simulink model "E_Platoon_simscape"  (R2025b)
settings: Solver=FixedStepAuto  StartTime=0.0  StopTime=inf  FixedStep=0.01  RelTol=1e-3
values from neighbouring files (symbols this model uses):
  battery_SOC_resistance = battery_SOC(:,3)    [EV_Truck.m]
  battery_SOC_SOC = battery_SOC(:,1)    [EV_Truck.m]
  battery_SOC_voltage = battery_SOC(:,2)    [EV_Truck.m]
  motor_efficiency_efficiency = table2array(motor_efficiency(2:height(motor_efficiency),2:width(motor_efficiency)))    [EV_Truck.m]
  motor_efficiency_RPM = table2array(motor_efficiency(2:height(motor_efficiency),1))    [EV_Truck.m]
  motor_efficiency_torque = transpose(motor_efficiency_torque)    [EV_Truck.m]
  motor_RPM_torque = table2array(motor_torque(1:14,1))    [EV_Truck.m]
  motor_torque_RPM = table2array(motor_torque(1:14,2))    [EV_Truck.m]
undefined symbols (not defined in the file or in its folder): battery_builder_rtmsupport, DiscIntNeverNeededParam, gcbh
libraries: simulink x8, fl_lib x8, nesl_utility x8, Batteries_lib x4, mpcadaslib x2, slpidlib x2
(part 1 of 3)
settings Model: Creator=Administrator  LastModifiedBy=geunu6319
settings SolverCC: AlgebraicLoopSolver=TrustRegion
settings DataIOCC: ExternalInput=EV_ModelingScenario.getElement('Input')  ReturnWorkspaceOutputs=off
settings OptimizationCC: DefaultParameterBehavior=Inlined  UseDivisionForNetSlopeComputation=on  GainParamInheritBuiltInType=on  UseFloatMulNetSlope=on  UseSpecifiedMinMax=on  InlineInvariantSignals=on  PassReuseOutputArgsAs=Individual arguments  ZeroExternalMemoryAtStartup=off  ZeroInternalMemoryAtStartup=off  NoFixptDivByZeroProtection=on  EfficientFloat2IntCast=on  LifeSpan=1  OptimizeBlockOrder=speed  DifferentSizesBufferReuse=on  EfficientTunableParamExpr=on
settings DebuggingCC: ParameterTunabilityLossMsg=error  UnconnectedInputMsg=warning  UnconnectedOutputMsg=warning  UnconnectedLineMsg=warning
settings HardwareCC: TargetBitPerLong=64.0  TargetBitPerPointer=64.0  TargetBitPerSizeT=64.0  TargetBitPerPtrDiffT=64.0  TargetLargestAtomicInteger=LongLong  TargetLargestAtomicFloat=Double  TargetLongLongMode=on  TargetIntDivRoundTo=Zero  TargetEndianess=LittleEndian  TargetWordSize=64.0  TargetHWDeviceType=ARM Compatible->ARM Cortex-A (64-bit)
settings ModelReferenceCC: EnableRefExpFcnMdlSchedulingChecks=on
settings SFSimCC: CompileTimeRecursionLimit=0.0  EnableRuntimeRecursion=off  MATLABDynamicMemAlloc=off  SimTargetLang=C++  SimDLTargetLibrary=mkl-dnn
settings RTWCC: SystemTargetFile=ert.tlc  GenCodeOnly=on  TemplateMakefile=ert_default_tmf  BuildConfiguration=Faster Runs  PortableWordSizes=on  CodeExecutionProfiling=on  CodeProfilingSaveOptions=AllData  CodeProfilingInstrumentation=coarse  DataTypeReplacement=CDataTypesFixedWidth  TargetLang=C++  GPUComputeCapability=3.5  DLArmComputeVersion=19.05  Description=Embedded Coder
settings CodeAppCC: ForceParamTrailComments=on  IgnoreCustomStorageClasses=off  IgnoreTestpoints=on  OperatorAnnotations=on  SimulinkDataObjDesc=on  SFDataObjDesc=on  CustomSymbolStrGlobalVar=rt$N$M  CustomSymbolStrType=$N$M  CustomSymbolStrFcn=$N$M$F  CustomSymbolStrMacro=$N$M  InsertBlockDesc=on
settings ERTTargetCC: RootIOFormat=Structure reference  ERTCustomFileTemplate=example_file_process.tlc  ERTFilePackagingFormat=CompactWithDataFile  SuppressUnreachableDefaultCases=off  MaxIdInt64=INT64_MAX  MinIdInt64=INT64_MIN  MaxIdUint64=UINT64_MAX  MaxIdInt32=INT32_MAX  MinIdInt32=INT32_MIN  MaxIdUint32=UINT32_MAX  MaxIdInt16=INT16_MAX  MinIdInt16=INT16_MIN  MaxIdUint16=UINT16_MAX  MaxIdInt8=INT8_MAX  MinIdInt8=INT8_MIN  MaxIdUint8=UINT8_MAX  TargetLangStandard=C++11 (ISO)  GenerateSampleERTMain=on  IncludeMdlTerminateFcn=off  CombineSignalStateStructs=on  CodeInterfacePackaging=C++ class  SupportComplex=off  SupportContinuousTime=on  SupportNonInlinedSFcns=on  ParenthesesLevel=Standards

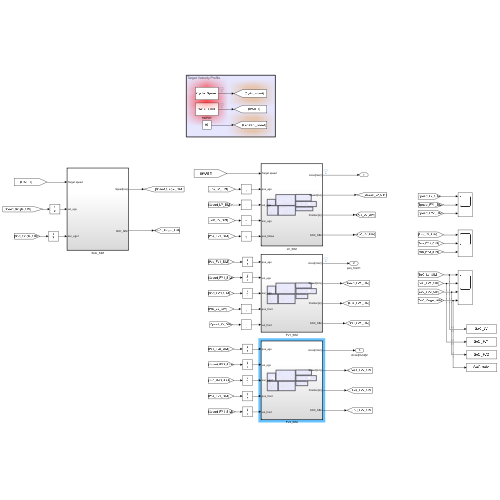
[thumbnail: Simulink's stored preview of the top-level diagram]
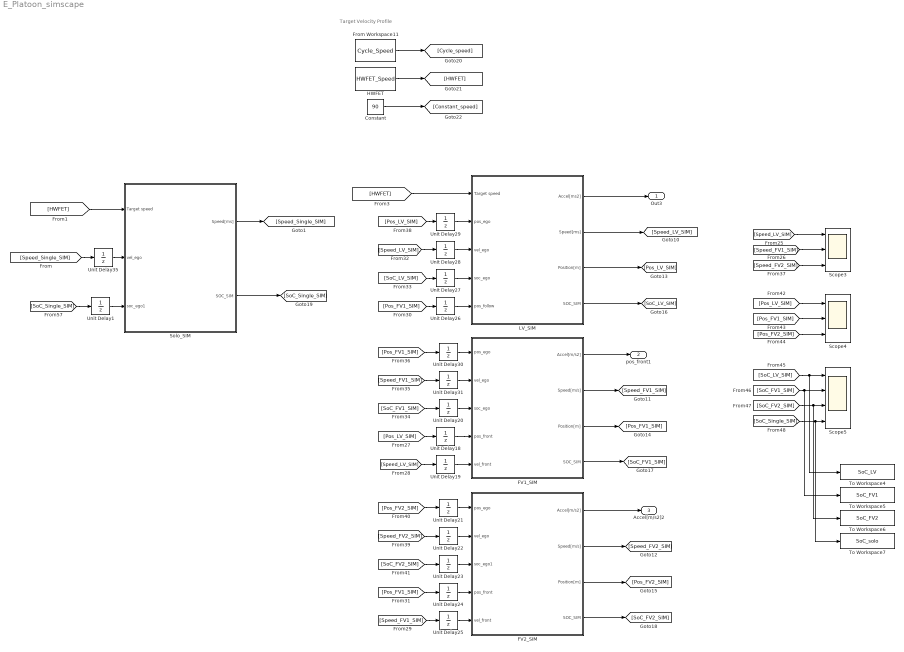
== system E_Platoon_simscape ==
  note: Target Velocity Profile
  Constant : Constant  Value=90  SampleTime=0.01
  FV1_SIM : Subsystem  TreatAsAtomicUnit=on
  FV2_SIM : Subsystem  TreatAsAtomicUnit=on
  From Workspace11 : FromWorkspace  VariableName=Cycle_Speed  SampleTime=0.01
  HWFET : FromWorkspace  VariableName=HWFET_Speed  SampleTime=0.01
  LV_SIM : Subsystem  TreatAsAtomicUnit=on
  Scope3 : Scope  NumInputPorts=3
      settings: ActiveDisplayYMinimum=-7.28265  ActiveDisplayYMaximum=34.73766
  Scope4 : Scope  NumInputPorts=3
      settings: ActiveDisplayYMinimum=-49042.71004  ActiveDisplayYMaximum=441032.69032  DataLoggingVariableName=ScopeData2
  Scope5 : Scope  NumInputPorts=4
      settings: ActiveDisplayYMinimum=92.43108  ActiveDisplayYMaximum=100.84099  DataLoggingVariableName=ScopeData3
  Solo_SIM : Subsystem  TreatAsAtomicUnit=on
  To Workspace4 : ToWorkspace  VariableName=SoC_LV  SaveFormat=Timeseries  SampleTime=-1
  To Workspace5 : ToWorkspace  VariableName=SoC_FV1  SaveFormat=Timeseries  SampleTime=-1
  To Workspace6 : ToWorkspace  VariableName=SoC_FV2  SaveFormat=Timeseries  SampleTime=-1
  To Workspace7 : ToWorkspace  VariableName=SoC_solo  SaveFormat=Timeseries  SampleTime=-1
  Unit Delay{1,18..31,35} (16 alike) : UnitDelay  SampleTime=-1  HasFrameUpgradeWarning=on
  Out3 : Outport
  pos_front1 : Outport  Port=2
  Accel[m/s2]2 : Outport  Port=3
  wires:
  Unit Delay35/1 -> Solo_SIM/2(vel_ego)
  [SoC_Single_SIM] -> Unit Delay1/1
  [HWFET] -> Solo_SIM/1(Target speed)
  Unit Delay27/1 -> LV_SIM/4(soc_ego)
  [SoC_LV_SIM] -> To Workspace4/1, Scope5/1
  [SoC_LV_SIM] -> Unit Delay27/1
  Unit Delay26/1 -> LV_SIM/5(pos_follow)
  Unit Delay24/1 -> FV2_SIM/4(pos_front)
  Unit Delay25/1 -> FV2_SIM/5(vel_front)
  [Speed_LV_SIM] -> Scope3/1
  [Pos_LV_SIM] -> Scope4/1
  Unit Delay28/1 -> LV_SIM/3(vel_ego)
  [SoC_FV2_SIM] -> To Workspace6/1, Scope5/3
  Unit Delay21/1 -> FV2_SIM/1(pos_ego)
  [HWFET] -> LV_SIM/1(Target speed)
  Unit Delay31/1 -> FV1_SIM/2(vel_ego)
  [Pos_FV1_SIM] -> Unit Delay26/1
  FV1_SIM/3(Position[m]) -> [Pos_FV1_SIM]
  [Speed_FV1_SIM] -> Unit Delay25/1
  [Pos_FV1_SIM] -> Scope4/2
  LV_SIM/3(Position[m]) -> [Pos_LV_SIM]
  [Pos_LV_SIM] -> Unit Delay29/1
  [Pos_FV1_SIM] -> Unit Delay30/1
  [SoC_FV1_SIM] -> To Workspace5/1, Scope5/2
  [Speed_FV2_SIM] -> Scope3/3
  FV2_SIM/2(Speed[m/s]) -> [Speed_FV2_SIM]
  FV1_SIM/4(SOC_SIM) -> [SoC_FV1_SIM]
  Unit Delay23/1 -> FV2_SIM/3(soc_ego1)
  Unit Delay22/1 -> FV2_SIM/2(vel_ego)
  [SoC_FV2_SIM] -> Unit Delay23/1
  [Speed_FV1_SIM] -> Unit Delay31/1
  [Speed_LV_SIM] -> Unit Delay19/1
  LV_SIM/2(Speed[ms]) -> [Speed_LV_SIM]
  FV2_SIM/3(Position[m]) -> [Pos_FV2_SIM]
  [SoC_FV1_SIM] -> Unit Delay20/1
  [Pos_FV2_SIM] -> Scope4/3
  [Speed_FV1_SIM] -> Scope3/2
  FV2_SIM/4(SOC_SIM) -> [SoC_FV2_SIM]
  LV_SIM/1(Accel[ms2]) -> Out3/1
  FV1_SIM/2(Speed[m/s]) -> [Speed_FV1_SIM]
  LV_SIM/4(SOC_SIM) -> [SoC_LV_SIM]
  [Pos_FV1_SIM] -> Unit Delay24/1
  [Speed_FV2_SIM] -> Unit Delay22/1
  [Speed_LV_SIM] -> Unit Delay28/1
  [Pos_FV2_SIM] -> Unit Delay21/1
  FV2_SIM/1(Accel[m/s2]) -> Accel[m/s2]2/1
  [SoC_Single_SIM] -> To Workspace7/1, Scope5/4
  Unit Delay30/1 -> FV1_SIM/1(pos_ego)
  [Pos_LV_SIM] -> Unit Delay18/1
  FV1_SIM/1(Accel[m/s2]) -> pos_front1/1
  Unit Delay29/1 -> LV_SIM/2(pos_ego)
  HWFET/1 -> [HWFET]
  From Workspace11/1 -> [Cycle_speed]
  Constant/1 -> [Constant_speed]
  Solo_SIM/2(SOC_SIM) -> [SoC_Single_SIM]
  Unit Delay20/1 -> FV1_SIM/3(soc_ego)
  Unit Delay18/1 -> FV1_SIM/4(pos_front)
  Unit Delay19/1 -> FV1_SIM/5(vel_front)
  Unit Delay1/1 -> Solo_SIM/3(soc_ego1)
  Solo_SIM/1(Speed[ms]) -> [Speed_Single_SIM]
  [Speed_Single_SIM] -> Unit Delay35/1

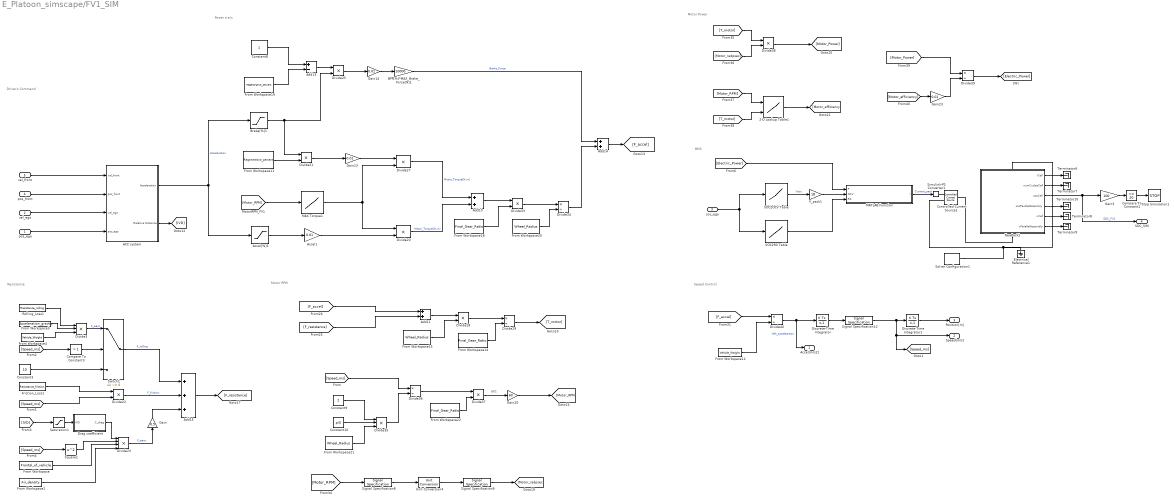
== system E_Platoon_simscape/FV1_SIM ==
  note: Driver's Command
  note: Motor RPM
  note: Motor Power
  note: Power train
  note: Speed Control
  note: RPS
  note: Resistance
  note: BMS
  pos_ego : Inport
  vel_ego : Inport  Port=2
  soc_ego : Inport  Port=3
  pos_front : Inport  Port=4
  vel_front : Inport  Port=5
  2-D Lookup Table1 : Lookup_n-D  BreakpointsForDimension1=motor_efficiency_RPM  BreakpointsForDimension2=motor_efficiency_torque  Table=motor_efficiency_efficiency  RemoveProtectionInput=on  InternalRulePriority=Speed  RndMeth=Simplest
      settings: InputPortMap=u0,u1
  ACC system : Subsystem
  Accel1 : Gain  Gain=0.01
  Accel[%]1 : Saturate  UpperLimit=100  LowerLimit=0
  Add10 : Sum
  Add11 : Sum
  Add13 : Sum  Inputs=+-
  Add14 : Sum
  Add15 : Sum  Inputs=+++
  BPP[%]*MAX_Brake_Force[N]1 : Gain  Gain=10000
  Brake[%]1 : Saturate  UpperLimit=0  LowerLimit=-100
  Compare To Constant1 : simulink/Logic and Bit Operations/Compare To Constant  relop=<=  const=20  OutDataTypeStr=boolean
  Compare To Constant3 : simulink/Logic and Bit Operations/Compare To Constant  relop=>  const=1  OutDataTypeStr=boolean
  Constant10 : Constant  Value=pi()
  Constant3 : Constant  Value=10
  Constant8 : Constant
  Constant9 : Constant  Value=2
  Controlled Current Source1 : fl_lib/Electrical/Electrical Sources/Controlled Current Source
  Discrete-Time Integrator : DiscreteIntegrator  SampleTime=-1  ICPrevOutput=DiscIntNeverNeededParam  ICPrevScaledInput=DiscIntNeverNeededParam
  Discrete-Time Integrator1 : DiscreteIntegrator  SampleTime=-1  ICPrevOutput=DiscIntNeverNeededParam  ICPrevScaledInput=DiscIntNeverNeededParam
  Divide{20..22,25,27..28,33,37..38} (9 alike) : Product  Inputs=**
  Divide23 : Product  Inputs=****
  Divide{29,34,36,39..40} (5 alike) : Product  Inputs=*/
  Divide3 : Product  Inputs=***
  Divide35 : Product  Inputs=***
  Drag coefficient : MATLAB Function  TreatAsAtomicUnit=on
  Electrical Reference1 : fl_lib/Electrical/Electrical Elements/Electrical Reference
  Friction_Loss1 : FromWorkspace  VariableName=Resistance_friction  SampleTime=0.01
  From Workspace : FromWorkspace  VariableName=Frontal_of_vehicle  SampleTime=0.01
  From Workspace11 : FromWorkspace  VariableName=Regenerative_percent  SampleTime=0.01
  From Workspace12 : FromWorkspace  VariableName=Vehicle_Weight  SampleTime=0.01
  From Workspace14 : FromWorkspace  VariableName=Final_Gear_Ratio  SampleTime=0.01
  From Workspace15 : FromWorkspace  VariableName=Wheel_Radius  SampleTime=0.01
  From Workspace18 : FromWorkspace  VariableName=Final_Gear_Ratio  SampleTime=0.01
  From Workspace19 : FromWorkspace  VariableName=Regenerative_percent  SampleTime=0.01
  From Workspace2 : FromWorkspace  VariableName=Air_density  SampleTime=0.01
  From Workspace20 : FromWorkspace  VariableName=Wheel_Radius  SampleTime=0.01
  From Workspace21 : FromWorkspace  VariableName=Wheel_Radius  SampleTime=0.01
  From Workspace22 : FromWorkspace  VariableName=Final_Gear_Ratio  SampleTime=0.01
  From Workspace3 : FromWorkspace  VariableName=Acceleration_gravity  SampleTime=0.01
  From Workspace4 : FromWorkspace  VariableName=Vehicle_Weight  SampleTime=0.01
  Gain : Gain  Gain=0.5
  Gain13 : Gain  Gain=0.01
  Gain14 : Gain  Gain=0.01
  Gain20 : Gain  Gain=60
  Gain23 : Gain  Gain=0.01
  Gain3 : Gain  Gain=100
  MATLAB Function : MATLAB Function  TreatAsAtomicUnit=on
  MAX Torque1 : Lookup_n-D  NumberOfTableDimensions=1  BreakpointsForDimension1=motor_RPM_torque  Table=motor_torque_RPM  RemoveProtectionInput=on  InternalRulePriority=Speed  RndMeth=Simplest
  NewPack1 : Subsystem  LoadFcn=battery_builder_rtmsupport('loadfcn',gcbh);
      settings: CopyFcn=battery_builder_rtmsupport('copyfcn',gcbh);  PreCopyFcn=battery_builder_rtmsupport('precopyfcn',gcbh);  PreDeleteFcn=battery_builder_rtmsupport('predeletefcn',gcbh);  PortSchema="{\"entries\":[{\"content\":{\"sides\":[{\"content\":{\"connectorIds\":[\"LConn1\"]},\"type\":\"ConnectorPlacement.EquallySpacedRectSide\",\"uuid\":\"1202e0a0-be56-4819-949f-0e575ff0fad5\"},{\"content\":{\"connectorIds\":[\"RConn1\"],\"side\":\"RIGHT\"},\"type\":\"ConnectorPlacement.EquallySpacedRectSide\",\"uuid\":\"c846b010-7318-4529-a495-49262266c279\"},{\"content\":{\"side\":\"TOP\"},\"type\":\"ConnectorPlacement.EquallySpacedRectSide\",\"uuid\":\"5cadc0b8-a7f2-47b4-97e8-4fab1bc2ac7d\"},{\"content\":{\"connectorIds\":[\"Out1\",\"Out2\",\"Out3\",\"Out4\",\"Out5\",\"Out6\"],\"side\":\"BOTTOM\"},\"type\":\"ConnectorPlacement.EquallySpacedRectSide\",\"uuid\":\"c5ce92ef-d0c0-4ddc-9166-c3c67527b5cc\"}]},\"type\":\"ConnectorPlacement.EquallySpacedConnector\",\"uuid\":\"4d056c7c-5936-459e-9daf-456b1978dca2\"}],\"packageUris\":[\"http://schema.mathworks.com/mf0/Connector/R2020b\"],\"version\":\"1.0\"}"
      mask Display: image('$imagefile')
  Rolling_Loss1 : FromWorkspace  VariableName=Resistance_rolling  SampleTime=0.01
  SOC2OCV Table : Lookup_n-D  NumberOfTableDimensions=1  BreakpointsForDimension1=battery_SOC_SOC  Table=battery_SOC_voltage  ExtrapMethod=Clip  RemoveProtectionInput=on  UseLastTableValue=on  InternalRulePriority=Speed  RndMeth=Simplest
  SOC2R0 Table : Lookup_n-D  NumberOfTableDimensions=1  BreakpointsForDimension1=battery_SOC_SOC  Table=battery_SOC_resistance  RemoveProtectionInput=on  InternalRulePriority=Speed  RndMeth=Simplest
  Saturation1 : Saturate  UpperLimit=100  LowerLimit=0
  Signal Specification12 : SignalSpecification  Unit=m/s
  Signal Specification8 : SignalSpecification  Unit=rpm
  Signal Specification9 : SignalSpecification  Unit=rad/s
  Simulink-PS Converter1 : nesl_utility/Simulink-PS Converter  PhysicalDomain=network_engine_domain  SubClassName=ps_input  LeftPortType=input  RightPortType=output  PseudoPeriodic=off  Frequencies=[]  NoiseDistribution=none  NoiseParameters=[]  Unit=1  AffineConversion=off  FilteringAndDerivatives=provide  SimscapeFilterOrder=1  InputFilterTimeConstant=0.001  UdotUserProvided=0
  Solver Configuration1 : nesl_utility/Solver Configuration  PhysicalDomain=network_engine_domain  SubClassName=solver  LeftPortType=input  RightPortType=generic  Tones=[]  Harmonics=[]  SimulateNoise=off  Profile=off  UseLocalSampling=off  EnableSwitchedLinearOptims=on  FrequencyDomain=off  UseCCode=off  RelTol=0.001  AbsTol=0.001  MinStep=1e-09  ToWorkspace=off  RevertToSquareIcSolve=off  NumHomotopyIterations=100  PhasorMode=off  PhasorModeNumHarmonics=1  ConsistencySolver=NEWTON_XTOL_AFTER_FTOL  IndexReductionMethod=DerivativeReplacement  DoDC=on  ResidualTolerance=1e-09  ConsistencyTolSource=GLOBAL  ConsistencyAbsTol=0.001  ConsistencyRelTol=0.001  ConsistencyTolFactor=0.001  UseLocalSolver=off  LocalSolverChoice=NE_BACKWARD_EULER_ADVANCER  ResolveIndetEquations=on  FunctionEvalNumThread=1  LocalSolverSampleTime=0.01  DoFixedCost=off  MaxNonlinIter=3  MaxModeIter=2  ComputeImpulses=off  ImpulseIterations=2  LinearAlgebra=auto  LinearAlgebraNumThread=0  EquationFormulation=NE_TIME_EF  DelaysMemoryBudget=1024  AutomaticFiltering=on  FilteringTimeConstant=0.001  PartitionStorageMethod=AS_NEEDED  PartitionMemoryBudget=1024  PartitionMethod=ROBUST  MultibodyUseLocalSolver=off  MultibodyLocalSolverChoice=ODE1  MultibodyLocalSolverSampleTime=0.001
  Square1 : Math  Operator=square
  Stop Simulation1 : Stop
  Switch1 : Switch  Criteria=u2 ~= 0  SaturateOnIntegerOverflow=off  InputSameDT=off
  Terminator{6..10} (5 alike) : Terminator
  Unit Conversion4 : UnitConversion
  V_pack1 : Gain  Gain=18
  Accel[m/s2] : Outport
  Speed[m/s] : Outport  Port=2
  Position[m] : Outport  Port=3
  SOC_SIM : Outport  Port=4
  wires:
  vel_front/1 -> ACC system/1(vel_front)
  pos_front/1 -> ACC system/2(pos_front)
  ACC system/2(Relative Distance) -> [IVD]
  From Workspace15/1 -> Divide28/2
  Divide28/1 -> Divide29/1
  From Workspace14/1 -> Divide29/2
  Divide37/1 -> Gain20/1
  Divide36/1 -> Divide37/1
  From Workspace21/1 -> Divide35/3
  Add10/1 -> Divide33/1
  Unit Conversion4/1 -> Signal Specification9/1
  Gain14/1 -> BPP[%]*MAX_Brake_Force[N]1/1
  Signal Specification9/1 -> [Motor_radpsec]
  MAX Torque1/1 -> Divide27/2, Divide20/1
  [Motor_RPM] -> MAX Torque1/1
  Divide35/1 -> Divide36/2
  [Motor_RPM] -> Signal Specification8/1
  Gain13/1 -> Divide27/1
  Divide39/1 -> [Electric_Power]
  Divide34/1 -> Add14/2
  Accel[%]1/1 -> Accel1/1
  [Motor_efficiency] -> Gain23/1
  Brake[%]1/1 -> Divide25/2, Divide21/1
  [Motor_RPM] -> 2-D Lookup Table1/1
  Divide25/1 -> Gain14/1
  Constant9/1 -> Divide35/1
  Add13/1 -> Divide25/1
  Divide20/1 -> Add10/2  "Motor_Torque[N.m]"
  [T_motor] -> Divide38/1
  Divide27/1 -> Add10/1  "Motor_Torque[N.m]"
  Divide33/1 -> Divide34/1
  Add14/1 -> [F_accel]
  From Workspace18/1 -> Divide33/2
  From Workspace20/1 -> Divide34/2
  BPP[%]*MAX_Brake_Force[N]1/1 -> Add14/1  "Brake_Force"
  Divide38/1 -> [Motor_Power]
  [F_accel] -> Add11/1
  Constant10/1 -> Divide35/2
  [Motor_Power] -> Divide39/1
  [Motor_radpsec] -> Divide38/2
  Gain20/1 -> [Motor_RPM]
  Divide21/1 -> Gain13/1
  [Speed_ms] -> Divide36/1
  Constant8/1 -> Add13/1
  Signal Specification8/1 -> Unit Conversion4/1
  Accel1/1 -> Divide20/2
  From Workspace19/1 -> Add13/2
  From Workspace11/1 -> Divide21/2
  2-D Lookup Table1/1 -> [Motor_efficiency]
  From Workspace22/1 -> Divide37/2
  Gain23/1 -> Divide39/2
  Divide29/1 -> [T_motor]
  [T_motor] -> 2-D Lookup Table1/2
  Add11/1 -> Divide28/1
  [F_resistance] -> Add11/2
  ACC system/1(Acceleration) -> Accel[%]1/1, Brake[%]1/1  "Acceleration"
  Divide40/1 -> Discrete-Time Integrator/1, Accel[m/s2]/1  "Veh_acceleartion"
  Discrete-Time Integrator1/1 -> Position[m]/1
  Signal Specification12/1 -> Discrete-Time Integrator1/1, [Speed_ms], Speed[m/s]/1
  From Workspace12/1 -> Divide40/2
  [F_accel] -> Divide40/1
  Discrete-Time Integrator/1 -> Signal Specification12/1
  From Workspace3/1 -> Divide3/2
  From Workspace/1 -> Divide23/3
  Gain/1 -> Add15/3
  From Workspace2/1 -> Divide23/4
  Divide3/1 -> Switch1/1  "F_aero"
  Divide23/1 -> Gain/1  "F_aero"
  From Workspace4/1 -> Divide3/3
  Saturation1/1 -> Drag coefficient/1(IVD)
  Add15/1 -> [F_resistance]
  Friction_Loss1/1 -> Divide22/1
  Drag coefficient/1(C_drag) -> Divide23/1
  Rolling_Loss1/1 -> Divide3/1
  Compare To Constant3/1 -> Switch1/2
  Square1/1 -> Divide23/2
  Constant3/1 -> Switch1/3
  [IVD] -> Saturation1/1
  [Speed_ms] -> Square1/1
  [Speed_ms] -> Divide22/2
  [Speed_ms] -> Compare To Constant3/1
  Divide22/1 -> Add15/2  "F_friction"
  Switch1/1 -> Add15/1  "F_rolling"
  pos_ego/1 -> ACC system/4(pos_ego)
  vel_ego/1 -> ACC system/3(vel_ego)
  NewPack1/5(vCell) -> Terminator8/1
  SOC2OCV Table/1 -> V_pack1/1  "Vsoc"
  SOC2R0 Table/1 -> MATLAB Function/3(R0)
  NewPack1/3(socCell) -> SOC_SIM/1, Gain3/1  "SOC_FV1"
  Compare To Constant1/1 -> Stop Simulation1/1
  NewPack1/4(socParallelAssembly) -> Terminator10/1
  Gain3/1 -> Compare To Constant1/1
  MATLAB Function/1(I) -> Simulink-PS Converter1/1  "Current_pack"
  NewPack1/2(numCyclesCell) -> Terminator7/1
  V_pack1/1 -> MATLAB Function/2(OCV)
  soc_ego/1 -> SOC2R0 Table/1, SOC2OCV Table/1
  NewPack1/6(vParallelAssembly) -> Terminator9/1
  [Electric_Power] -> MATLAB Function/1(P)
  NewPack1/1(iCell) -> Terminator6/1
  connections:
  Solver Configuration1/RConn1 -- Controlled Current Source1/RConn2 -- Electrical Reference1/LConn1 -- NewPack1/LConn1
  Simulink-PS Converter1/RConn1 -- Controlled Current Source1/RConn1
  NewPack1/RConn1 -- Controlled Current Source1/LConn1

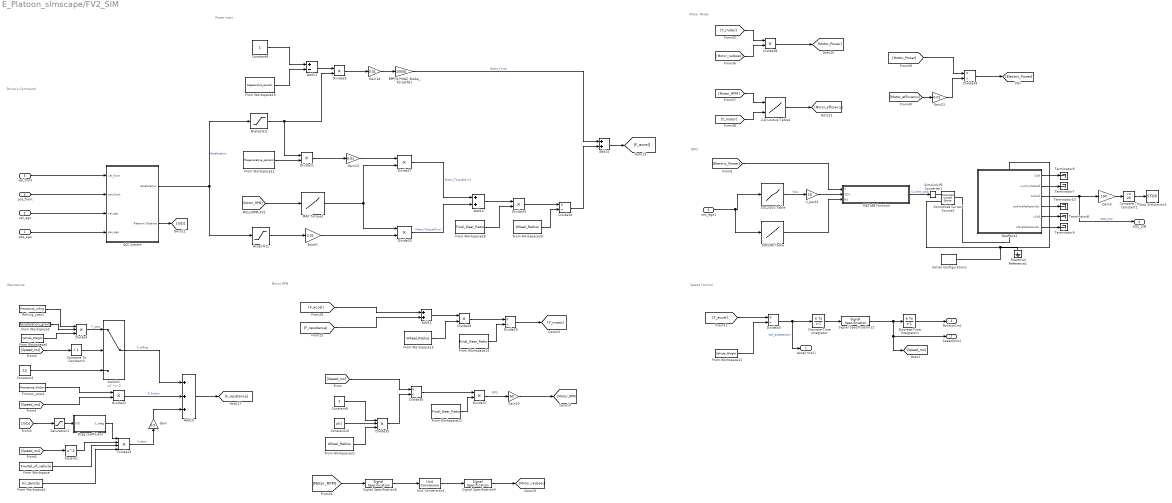
== system E_Platoon_simscape/FV2_SIM ==
  note: Driver's Command
  note: Motor RPM
  note: Motor Power
  note: Power train
  note: Speed Control
  note: RPS
  note: Resistance
  note: BMS
  pos_ego : Inport
  vel_ego : Inport  Port=2
  soc_ego1 : Inport  Port=3
  pos_front : Inport  Port=4
  vel_front : Inport  Port=5
  2-D Lookup Table1 : Lookup_n-D  BreakpointsForDimension1=motor_efficiency_RPM  BreakpointsForDimension2=motor_efficiency_torque  Table=motor_efficiency_efficiency  RemoveProtectionInput=on  InternalRulePriority=Speed  RndMeth=Simplest
      settings: InputPortMap=u0,u1
  ACC system : Subsystem
  Accel1 : Gain  Gain=0.01
  Accel[%]1 : Saturate  UpperLimit=100  LowerLimit=0
  Add10 : Sum
  Add11 : Sum
  Add13 : Sum  Inputs=+-
  Add14 : Sum
  Add15 : Sum  Inputs=+++
  BPP[%]*MAX_Brake_Force[N]1 : Gain  Gain=10000
  Brake[%]1 : Saturate  UpperLimit=0  LowerLimit=-100
  Compare To Constant1 : simulink/Logic and Bit Operations/Compare To Constant  relop=<=  const=20  OutDataTypeStr=boolean
  Compare To Constant3 : simulink/Logic and Bit Operations/Compare To Constant  relop=>  const=1  OutDataTypeStr=boolean
  Constant10 : Constant  Value=pi()
  Constant3 : Constant  Value=10
  Constant8 : Constant
  Constant9 : Constant  Value=2
  Controlled Current Source1 : fl_lib/Electrical/Electrical Sources/Controlled Current Source
  Discrete-Time Integrator : DiscreteIntegrator  SampleTime=-1  ICPrevOutput=DiscIntNeverNeededParam  ICPrevScaledInput=DiscIntNeverNeededParam
  Discrete-Time Integrator1 : DiscreteIntegrator  SampleTime=-1  ICPrevOutput=DiscIntNeverNeededParam  ICPrevScaledInput=DiscIntNeverNeededParam
  Divide{20..22,25,27..28,33,37..38} (9 alike) : Product  Inputs=**
  Divide23 : Product  Inputs=****
  Divide{29,34,36,39..40} (5 alike) : Product  Inputs=*/
  Divide3 : Product  Inputs=***
  Divide35 : Product  Inputs=***
  Drag coefficient : MATLAB Function  TreatAsAtomicUnit=on
  Electrical Reference1 : fl_lib/Electrical/Electrical Elements/Electrical Reference
  Friction_Loss1 : FromWorkspace  VariableName=Resistance_friction  SampleTime=0.01
  From Workspace : FromWorkspace  VariableName=Frontal_of_vehicle  SampleTime=0.01
  From Workspace11 : FromWorkspace  VariableName=Regenerative_percent  SampleTime=0.01
  From Workspace12 : FromWorkspace  VariableName=Vehicle_Weight  SampleTime=0.01
  From Workspace14 : FromWorkspace  VariableName=Final_Gear_Ratio  SampleTime=0.01
  From Workspace15 : FromWorkspace  VariableName=Wheel_Radius  SampleTime=0.01
  From Workspace18 : FromWorkspace  VariableName=Final_Gear_Ratio  SampleTime=0.01
  From Workspace19 : FromWorkspace  VariableName=Regenerative_percent  SampleTime=0.01
  From Workspace2 : FromWorkspace  VariableName=Air_density  SampleTime=0.01
  From Workspace20 : FromWorkspace  VariableName=Wheel_Radius  SampleTime=0.01
  From Workspace21 : FromWorkspace  VariableName=Wheel_Radius  SampleTime=0.01
  From Workspace22 : FromWorkspace  VariableName=Final_Gear_Ratio  SampleTime=0.01
  From Workspace3 : FromWorkspace  VariableName=Acceleration_gravity  SampleTime=0.01
  From Workspace4 : FromWorkspace  VariableName=Vehicle_Weight  SampleTime=0.01
  Gain : Gain  Gain=0.5
  Gain13 : Gain  Gain=0.01
  Gain14 : Gain  Gain=0.01
  Gain20 : Gain  Gain=60
  Gain23 : Gain  Gain=0.01
  Gain3 : Gain  Gain=100
  MATLAB Function : MATLAB Function  TreatAsAtomicUnit=on
  MAX Torque1 : Lookup_n-D  NumberOfTableDimensions=1  BreakpointsForDimension1=motor_RPM_torque  Table=motor_torque_RPM  RemoveProtectionInput=on  InternalRulePriority=Speed  RndMeth=Simplest
  NewPack1 : Subsystem  LoadFcn=battery_builder_rtmsupport('loadfcn',gcbh);
      settings: CopyFcn=battery_builder_rtmsupport('copyfcn',gcbh);  PreCopyFcn=battery_builder_rtmsupport('precopyfcn',gcbh);  PreDeleteFcn=battery_builder_rtmsupport('predeletefcn',gcbh);  PortSchema="{\"entries\":[{\"content\":{\"sides\":[{\"content\":{\"connectorIds\":[\"LConn1\"]},\"type\":\"ConnectorPlacement.EquallySpacedRectSide\",\"uuid\":\"1202e0a0-be56-4819-949f-0e575ff0fad5\"},{\"content\":{\"connectorIds\":[\"RConn1\"],\"side\":\"RIGHT\"},\"type\":\"ConnectorPlacement.EquallySpacedRectSide\",\"uuid\":\"c846b010-7318-4529-a495-49262266c279\"},{\"content\":{\"side\":\"TOP\"},\"type\":\"ConnectorPlacement.EquallySpacedRectSide\",\"uuid\":\"5cadc0b8-a7f2-47b4-97e8-4fab1bc2ac7d\"},{\"content\":{\"connectorIds\":[\"Out1\",\"Out2\",\"Out3\",\"Out4\",\"Out5\",\"Out6\"],\"side\":\"BOTTOM\"},\"type\":\"ConnectorPlacement.EquallySpacedRectSide\",\"uuid\":\"c5ce92ef-d0c0-4ddc-9166-c3c67527b5cc\"}]},\"type\":\"ConnectorPlacement.EquallySpacedConnector\",\"uuid\":\"4d056c7c-5936-459e-9daf-456b1978dca2\"}],\"packageUris\":[\"http://schema.mathworks.com/mf0/Connector/R2020b\"],\"version\":\"1.0\"}"
      mask Display: image('$imagefile')
  Rolling_Loss1 : FromWorkspace  VariableName=Resistance_rolling  SampleTime=0.01
  SOC2OCV Table : Lookup_n-D  NumberOfTableDimensions=1  BreakpointsForDimension1=battery_SOC_SOC  Table=battery_SOC_voltage  ExtrapMethod=Clip  RemoveProtectionInput=on  UseLastTableValue=on  InternalRulePriority=Speed  RndMeth=Simplest
  SOC2R0 Table : Lookup_n-D  NumberOfTableDimensions=1  BreakpointsForDimension1=battery_SOC_SOC  Table=battery_SOC_resistance  RemoveProtectionInput=on  InternalRulePriority=Speed  RndMeth=Simplest
  Saturation1 : Saturate  UpperLimit=100  LowerLimit=0
  Signal Specification12 : SignalSpecification  Unit=m/s
  Signal Specification8 : SignalSpecification  Unit=rpm
  Signal Specification9 : SignalSpecification  Unit=rad/s
  Simulink-PS Converter1 : nesl_utility/Simulink-PS Converter  PhysicalDomain=network_engine_domain  SubClassName=ps_input  LeftPortType=input  RightPortType=output  PseudoPeriodic=off  Frequencies=[]  NoiseDistribution=none  NoiseParameters=[]  Unit=1  AffineConversion=off  FilteringAndDerivatives=provide  SimscapeFilterOrder=1  InputFilterTimeConstant=0.001  UdotUserProvided=0
  Solver Configuration1 : nesl_utility/Solver Configuration  PhysicalDomain=network_engine_domain  SubClassName=solver  LeftPortType=input  RightPortType=generic  Tones=[]  Harmonics=[]  SimulateNoise=off  Profile=off  UseLocalSampling=off  EnableSwitchedLinearOptims=on  FrequencyDomain=off  UseCCode=off  RelTol=0.001  AbsTol=0.001  MinStep=1e-09  ToWorkspace=off  RevertToSquareIcSolve=off  NumHomotopyIterations=100  PhasorMode=off  PhasorModeNumHarmonics=1  ConsistencySolver=NEWTON_XTOL_AFTER_FTOL  IndexReductionMethod=DerivativeReplacement  DoDC=on  ResidualTolerance=1e-09  ConsistencyTolSource=GLOBAL  ConsistencyAbsTol=0.001  ConsistencyRelTol=0.001  ConsistencyTolFactor=0.001  UseLocalSolver=off  LocalSolverChoice=NE_BACKWARD_EULER_ADVANCER  ResolveIndetEquations=on  FunctionEvalNumThread=1  LocalSolverSampleTime=0.01  DoFixedCost=off  MaxNonlinIter=3  MaxModeIter=2  ComputeImpulses=off  ImpulseIterations=2  LinearAlgebra=auto  LinearAlgebraNumThread=0  EquationFormulation=NE_TIME_EF  DelaysMemoryBudget=1024  AutomaticFiltering=on  FilteringTimeConstant=0.001  PartitionStorageMethod=AS_NEEDED  PartitionMemoryBudget=1024  PartitionMethod=ROBUST  MultibodyUseLocalSolver=off  MultibodyLocalSolverChoice=ODE1  MultibodyLocalSolverSampleTime=0.001
  Square1 : Math  Operator=square
  Stop Simulation1 : Stop
  Switch1 : Switch  Criteria=u2 ~= 0  SaturateOnIntegerOverflow=off  InputSameDT=off
  Terminator{6..10} (5 alike) : Terminator
  Unit Conversion4 : UnitConversion
  V_pack1 : Gain  Gain=18
  Accel[m/s2] : Outport
  Speed[m/s] : Outport  Port=2
  Position[m] : Outport  Port=3
  SOC_SIM : Outport  Port=4
  wires:
  vel_front/1 -> ACC system/1(vel_front)
  pos_front/1 -> ACC system/2(pos_front)
  ACC system/2(Relative Distance) -> [IVD]
  From Workspace15/1 -> Divide28/2
  Divide28/1 -> Divide29/1
  From Workspace14/1 -> Divide29/2
  Divide37/1 -> Gain20/1
  Divide36/1 -> Divide37/1
  From Workspace21/1 -> Divide35/3
  Add10/1 -> Divide33/1
  Unit Conversion4/1 -> Signal Specification9/1
  Gain14/1 -> BPP[%]*MAX_Brake_Force[N]1/1
  Signal Specification9/1 -> [Motor_radpsec]
  MAX Torque1/1 -> Divide27/2, Divide20/1
  [Motor_RPM] -> MAX Torque1/1
  Divide35/1 -> Divide36/2
  [Motor_RPM] -> Signal Specification8/1
  Gain13/1 -> Divide27/1
  Divide39/1 -> [Electric_Power]
  Divide34/1 -> Add14/2
  Accel[%]1/1 -> Accel1/1
  [Motor_efficiency] -> Gain23/1
  Brake[%]1/1 -> Divide25/2, Divide21/1
  [Motor_RPM] -> 2-D Lookup Table1/1
  Divide25/1 -> Gain14/1
  Constant9/1 -> Divide35/1
  Add13/1 -> Divide25/1
  Divide20/1 -> Add10/2  "Motor_Torque[N.m]"
  [T_motor] -> Divide38/1
  Divide27/1 -> Add10/1  "Motor_Torque[N.m]"
  Divide33/1 -> Divide34/1
  Add14/1 -> [F_accel]
  From Workspace18/1 -> Divide33/2
  From Workspace20/1 -> Divide34/2
  BPP[%]*MAX_Brake_Force[N]1/1 -> Add14/1  "Brake_Force"
  Divide38/1 -> [Motor_Power]
  [F_accel] -> Add11/1
  Constant10/1 -> Divide35/2
  [Motor_Power] -> Divide39/1
  [Motor_radpsec] -> Divide38/2
  Gain20/1 -> [Motor_RPM]
  Divide21/1 -> Gain13/1
  [Speed_ms] -> Divide36/1
  Constant8/1 -> Add13/1
  Signal Specification8/1 -> Unit Conversion4/1
  Accel1/1 -> Divide20/2
  From Workspace19/1 -> Add13/2
  From Workspace11/1 -> Divide21/2
  2-D Lookup Table1/1 -> [Motor_efficiency]
  From Workspace22/1 -> Divide37/2
  Gain23/1 -> Divide39/2
  Divide29/1 -> [T_motor]
  [T_motor] -> 2-D Lookup Table1/2
  Add11/1 -> Divide28/1
  [F_resistance] -> Add11/2
  ACC system/1(Acceleration) -> Accel[%]1/1, Brake[%]1/1  "Acceleration"
  Divide40/1 -> Discrete-Time Integrator/1, Accel[m/s2]/1  "Veh_acceleartion"
  Discrete-Time Integrator1/1 -> Position[m]/1
  Signal Specification12/1 -> Discrete-Time Integrator1/1, [Speed_ms], Speed[m/s]/1
  From Workspace12/1 -> Divide40/2
  [F_accel] -> Divide40/1
  Discrete-Time Integrator/1 -> Signal Specification12/1
  From Workspace3/1 -> Divide3/2
  From Workspace/1 -> Divide23/3
  Gain/1 -> Add15/3
  From Workspace2/1 -> Divide23/4
  Divide3/1 -> Switch1/1  "F_aero"
  Divide23/1 -> Gain/1  "F_aero"
  From Workspace4/1 -> Divide3/3
  Saturation1/1 -> Drag coefficient/1(IVD)
  Add15/1 -> [F_resistance]
  Friction_Loss1/1 -> Divide22/1
  Drag coefficient/1(C_drag) -> Divide23/1
  Rolling_Loss1/1 -> Divide3/1
  Compare To Constant3/1 -> Switch1/2
  Square1/1 -> Divide23/2
  Constant3/1 -> Switch1/3
  [IVD] -> Saturation1/1
  [Speed_ms] -> Square1/1
  [Speed_ms] -> Divide22/2
  [Speed_ms] -> Compare To Constant3/1
  Divide22/1 -> Add15/2  "F_friction"
  Switch1/1 -> Add15/1  "F_rolling"
  pos_ego/1 -> ACC system/4(pos_ego)
  vel_ego/1 -> ACC system/3(vel_ego)
  NewPack1/5(vCell) -> Terminator8/1
  SOC2OCV Table/1 -> V_pack1/1  "Vsoc"
  SOC2R0 Table/1 -> MATLAB Function/3(R0)
  NewPack1/3(socCell) -> SOC_SIM/1, Gain3/1  "SOC_FV2"
  Compare To Constant1/1 -> Stop Simulation1/1
  NewPack1/4(socParallelAssembly) -> Terminator10/1
  Gain3/1 -> Compare To Constant1/1
  MATLAB Function/1(I) -> Simulink-PS Converter1/1  "Current_pack"
  NewPack1/2(numCyclesCell) -> Terminator7/1
  V_pack1/1 -> MATLAB Function/2(OCV)
  soc_ego1/1 -> SOC2R0 Table/1, SOC2OCV Table/1
  NewPack1/6(vParallelAssembly) -> Terminator9/1
  [Electric_Power] -> MATLAB Function/1(P)
  NewPack1/1(iCell) -> Terminator6/1
  connections:
  Solver Configuration1/RConn1 -- Controlled Current Source1/RConn2 -- Electrical Reference1/LConn1 -- NewPack1/LConn1
  Simulink-PS Converter1/RConn1 -- Controlled Current Source1/RConn1
  NewPack1/RConn1 -- Controlled Current Source1/LConn1

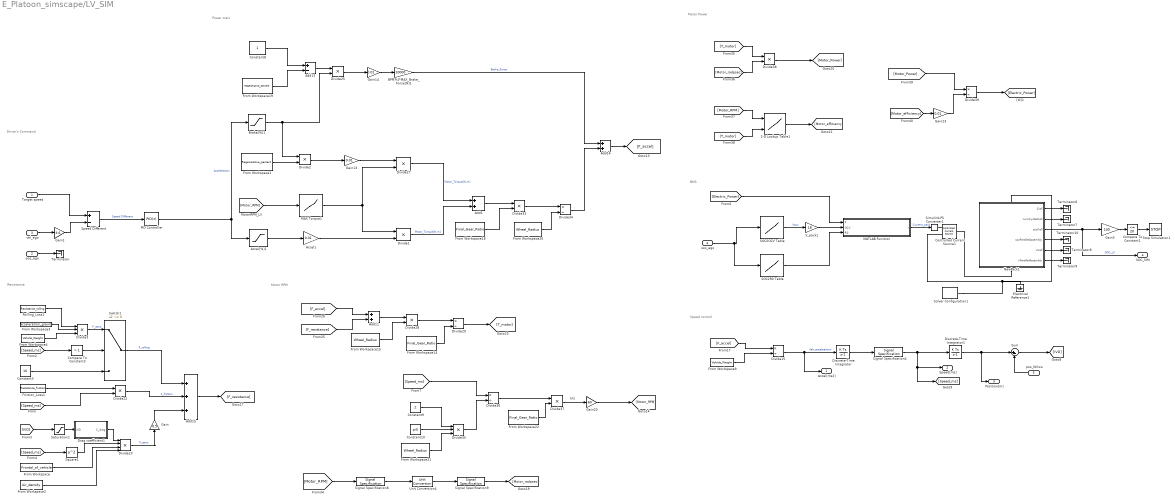
== system E_Platoon_simscape/LV_SIM ==
  note: Speed control
  note: Driver's Command
  note: RPS
  note: Power train
  note: Resistance
  note: Motor RPM
  note: Motor Power
  note: BMS
  Target speed : Inport
  pos_ego : Inport  Port=2
  vel_ego : Inport  Port=3
  soc_ego : Inport  Port=4
  pos_follow : Inport  Port=5
  2-D Lookup Table1 : Lookup_n-D  BreakpointsForDimension1=motor_efficiency_RPM  BreakpointsForDimension2=motor_efficiency_torque  Table=motor_efficiency_efficiency  InternalRulePriority=Speed  RndMeth=Simplest
      settings: InputPortMap=u0,u1
  Accel1 : Gain  Gain=0.01
  Accel[%]1 : Saturate  UpperLimit=100  LowerLimit=0
  Add1 : Sum
  Add11 : Sum
  Add13 : Sum  Inputs=+-
  Add14 : Sum
  Add15 : Sum  Inputs=+++
  BPP[%]*MAX_Brake_Force[N]1 : Gain  Gain=10000
  Brake[%]1 : Saturate  UpperLimit=0  LowerLimit=-100
  Compare To Constant1 : simulink/Logic and Bit Operations/Compare To Constant  relop=<=  const=20  OutDataTypeStr=boolean
  Compare To Constant3 : simulink/Logic and Bit Operations/Compare To Constant  relop=>  const=1  OutDataTypeStr=boolean
  Constant10 : Constant  Value=pi()
  Constant3 : Constant  Value=10
  Constant8 : Constant
  Constant9 : Constant  Value=2
  Controlled Current Source1 : fl_lib/Electrical/Electrical Sources/Controlled Current Source
  Discrete-Time Integrator : DiscreteIntegrator  SampleTime=-1  ICPrevOutput=DiscIntNeverNeededParam  ICPrevScaledInput=DiscIntNeverNeededParam
  Discrete-Time Integrator1 : DiscreteIntegrator  SampleTime=-1  ICPrevOutput=DiscIntNeverNeededParam  ICPrevScaledInput=DiscIntNeverNeededParam
  Divide{1..2,22,25,27..28,33,37..38} (9 alike) : Product  Inputs=**
  Divide{15,29,34,36,39} (5 alike) : Product  Inputs=*/
  Divide23 : Product  Inputs=****
  Divide3 : Product  Inputs=***
  Divide35 : Product  Inputs=***
  Drag coefficient1 : MATLAB Function  TreatAsAtomicUnit=on
  Electrical Reference1 : fl_lib/Electrical/Electrical Elements/Electrical Reference
  Friction_Loss1 : FromWorkspace  VariableName=Resistance_friction  SampleTime=0.01
  From Workspace : FromWorkspace  VariableName=Frontal_of_vehicle  SampleTime=0.01
  From Workspace1 : FromWorkspace  VariableName=Regenerative_percent  SampleTime=0.01
  From Workspace14 : FromWorkspace  VariableName=Final_Gear_Ratio  SampleTime=0.01
  From Workspace15 : FromWorkspace  VariableName=Wheel_Radius  SampleTime=0.01
  From Workspace18 : FromWorkspace  VariableName=Final_Gear_Ratio  SampleTime=0.01
  From Workspace19 : FromWorkspace  VariableName=Regenerative_percent  SampleTime=0.01
  From Workspace2 : FromWorkspace  VariableName=Air_density  SampleTime=0.01
  From Workspace20 : FromWorkspace  VariableName=Wheel_Radius  SampleTime=0.01
  From Workspace21 : FromWorkspace  VariableName=Wheel_Radius  SampleTime=0.01
  From Workspace22 : FromWorkspace  VariableName=Final_Gear_Ratio  SampleTime=0.01
  From Workspace3 : FromWorkspace  VariableName=Acceleration_gravity  SampleTime=0.01
  From Workspace4 : FromWorkspace  VariableName=Vehicle_Weight  SampleTime=0.01
  From Workspace9 : FromWorkspace  VariableName=Vehicle_Weight  SampleTime=0.01
  Gain : Gain  Gain=0.5
  Gain1 : Gain  Gain=3.6
  Gain13 : Gain  Gain=0.01
  Gain14 : Gain  Gain=0.01
  Gain20 : Gain  Gain=60
  Gain23 : Gain  Gain=0.01
  Gain3 : Gain  Gain=100
  MATLAB Function : MATLAB Function  TreatAsAtomicUnit=on
  MAX Torque1 : Lookup_n-D  NumberOfTableDimensions=1  BreakpointsForDimension1=motor_RPM_torque  Table=motor_torque_RPM  InternalRulePriority=Speed  RndMeth=Simplest
  NewPack1 : Subsystem  LoadFcn=battery_builder_rtmsupport('loadfcn',gcbh);
      settings: CopyFcn=battery_builder_rtmsupport('copyfcn',gcbh);  PreCopyFcn=battery_builder_rtmsupport('precopyfcn',gcbh);  PreDeleteFcn=battery_builder_rtmsupport('predeletefcn',gcbh);  PortSchema="{\"entries\":[{\"content\":{\"sides\":[{\"content\":{\"connectorIds\":[\"LConn1\"]},\"type\":\"ConnectorPlacement.EquallySpacedRectSide\",\"uuid\":\"1202e0a0-be56-4819-949f-0e575ff0fad5\"},{\"content\":{\"connectorIds\":[\"RConn1\"],\"side\":\"RIGHT\"},\"type\":\"ConnectorPlacement.EquallySpacedRectSide\",\"uuid\":\"c846b010-7318-4529-a495-49262266c279\"},{\"content\":{\"side\":\"TOP\"},\"type\":\"ConnectorPlacement.EquallySpacedRectSide\",\"uuid\":\"5cadc0b8-a7f2-47b4-97e8-4fab1bc2ac7d\"},{\"content\":{\"connectorIds\":[\"Out1\",\"Out2\",\"Out3\",\"Out4\",\"Out5\",\"Out6\"],\"side\":\"BOTTOM\"},\"type\":\"ConnectorPlacement.EquallySpacedRectSide\",\"uuid\":\"c5ce92ef-d0c0-4ddc-9166-c3c67527b5cc\"}]},\"type\":\"ConnectorPlacement.EquallySpacedConnector\",\"uuid\":\"4d056c7c-5936-459e-9daf-456b1978dca2\"}],\"packageUris\":[\"http://schema.mathworks.com/mf0/Connector/R2020b\"],\"version\":\"1.0\"}"
      mask Display: image('$imagefile')
  PID Controller : slpidlib/PID Controller  Controller=PID  Form=Parallel  TimeDomain=Discrete-time  UseExternalTs=off  SampleTime=0.01  IntegratorMethod=Forward Euler  FilterMethod=Forward Euler  ControllerParametersSource=internal  P=100  I=0.01  UseKiTs=off  D=0.0001  UseExternalDerivativeSource=off  N=10  UseFilter=on  TunerSelectOption=Transfer Function Based (PID Tuner App)  InitialConditionSource=internal  InitialConditionForIntegrator=0  InitialConditionForFilter=0  DifferentiatorICPrevScaledInput=0  ExternalReset=none  TrackingMode=off  Kt=1  LimitOutput=off  SatLimitsSource=internal  UpperSaturationLimit=inf  LowerSaturationLimit=-inf  LinearizeAsGain=on  AntiWindupMode=none  Kb=1  LimitIntegrator=off  UpperIntegratorSaturationLimit=inf  LowerIntegratorSaturationLimit=-inf  POutMin=[]  POutMax=[]  IOutMin=[]  IOutMax=[]  DOutMin=[]  DOutMax=[]  NOutMin=[]  NOutMax=[]  SumOutMin=[]  SumOutMax=[]  SaturationOutMin=[]  SaturationOutMax=[]  PParamMin=[]  PParamMax=[]  IParamMin=[]  IParamMax=[]  DParamMin=[]  DParamMax=[]  NParamMin=[]  NParamMax=[]  KbParamMin=[]  KbParamMax=[]  KtParamMin=[]  KtParamMax=[]  KbOutMin=[]  KbOutMax=[]  KtOutMin=[]  KtOutMax=[]  IntegratorOutMin=[]  IntegratorOutMax=[]  FilterOutMin=[]  FilterOutMax=[]  SumI1OutMin=[]  SumI1OutMax=[]  SumI2OutMin=[]  SumI2OutMax=[]  SumI3OutMin=[]  SumI3OutMax=[]  SumI4OutMin=[]  SumI4OutMax=[]  SumDOutMin=[]  SumDOutMax=[]  DifferentiatorOutMin=[]  DifferentiatorOutMax=[]  FilterDiffOutCoefMin=[]  FilterDiffOutCoefMax=[]  ReciprocalOutMin=[]  ReciprocalOutMax=[]  SumDenOutMin=[]  SumDenOutMax=[]  SumNumOutMin=[]  SumNumOutMax=[]  DivideOutMin=[]  DivideOutMax=[]  UdiffTsProdOutMin=[]  UdiffTsProdOutMax=[]  NTsProdOutMin=[]  NTsProdOutMax=[]  UintegralTsProdOutMin=[]  UintegralTsProdOutMax=[]  UngainTsProdOutMin=[]  UngainTsProdOutMax=[]  ClampingZeroOutDataTypeStr=Inherit: Inherit via back propagation  ClampingZeroOutMin=[]  ClampingZeroOutMax=[]  FilterDenConstantOutDataTypeStr=Inherit: Inherit via back propagation  FilterDenConstantOutMin=[]  FilterDenConstantOutMax=[]  PCopyOutDataTypeStr=Inherit: Inherit via back propagation  PCopyOutMin=[]  PCopyOutMax=[]  NCopyOutDataTypeStr=Inherit: Inherit via back propagation  NCopyOutMin=[]  NCopyOutMax=[]  IntegratorContinuousStateAttributes=''  IntegratorStateMustResolveToSignalObject=off  IntegratorRTWStateStorageClass=Auto  FilterContinuousStateAttributes=''  FilterStateMustResolveToSignalObject=off  FilterRTWStateStorageClass=Auto  ParallelPVariant=InternalParameters  IdealPVariant=Disabled  IVariant=InternalParameters  DVariant=InternalParameters  IntegratorVariant=Discrete  SatVariant=Disabled  AWVariant=Passthrough  PCopyVariant=Disabled  TRVariant=Disabled  FdbkBlocksVariant=Forward  IdealPFdbkVariant=Disabled  SatFdbkVariant=Disabled  DerivativeFilterVariant=ForwardEulerFilter  NVariant=InternalParameters  NCopyVariant=Disabled  FilterICVariant=InternalICsFilter  IntegratorICVariant=InternalICs  ExternalResetVariant=Disabled  TRSumVariant=Passthrough  SumFdbkVariant=Disabled  SumVariant=Sum_PID  TsampFilterVariant=InternalTs  TsampNgainVariant=Passthrough  TsampIntegralVariant=Disabled_SignalSpec  ExternalSaturationOutDataTypeStr=Inherit: Same as second input  DerivativeSourceVariant=ErrorSignal  PreIntVariant=InternalPreInt
  Rolling_Loss1 : FromWorkspace  VariableName=Resistance_rolling  SampleTime=0.01
  SOC2OCV Table : Lookup_n-D  NumberOfTableDimensions=1  BreakpointsForDimension1=battery_SOC_SOC  Table=battery_SOC_voltage  ExtrapMethod=Clip  RemoveProtectionInput=on  UseLastTableValue=on  InternalRulePriority=Speed  RndMeth=Simplest
  SOC2R0 Table : Lookup_n-D  NumberOfTableDimensions=1  BreakpointsForDimension1=battery_SOC_SOC  Table=battery_SOC_resistance  RemoveProtectionInput=on  InternalRulePriority=Speed  RndMeth=Simplest
  Saturation1 : Saturate  UpperLimit=100  LowerLimit=0
  Signal Specification4 : SignalSpecification  Unit=m/s
  Signal Specification8 : SignalSpecification  Unit=rpm
  Signal Specification9 : SignalSpecification  Unit=rad/s
  Simulink-PS Converter1 : nesl_utility/Simulink-PS Converter  PhysicalDomain=network_engine_domain  SubClassName=ps_input  LeftPortType=input  RightPortType=output  PseudoPeriodic=off  Frequencies=[]  NoiseDistribution=none  NoiseParameters=[]  Unit=1  AffineConversion=off  FilteringAndDerivatives=provide  SimscapeFilterOrder=1  InputFilterTimeConstant=0.001  UdotUserProvided=0
  Solver Configuration1 : nesl_utility/Solver Configuration  PhysicalDomain=network_engine_domain  SubClassName=solver  LeftPortType=input  RightPortType=generic  Tones=[]  Harmonics=[]  SimulateNoise=off  Profile=off  UseLocalSampling=off  EnableSwitchedLinearOptims=on  FrequencyDomain=off  UseCCode=off  RelTol=0.001  AbsTol=0.001  MinStep=1e-09  ToWorkspace=off  RevertToSquareIcSolve=off  NumHomotopyIterations=100  PhasorMode=off  PhasorModeNumHarmonics=1  ConsistencySolver=NEWTON_XTOL_AFTER_FTOL  IndexReductionMethod=DerivativeReplacement  DoDC=on  ResidualTolerance=1e-09  ConsistencyTolSource=GLOBAL  ConsistencyAbsTol=0.001  ConsistencyRelTol=0.001  ConsistencyTolFactor=0.001  UseLocalSolver=off  LocalSolverChoice=NE_BACKWARD_EULER_ADVANCER  ResolveIndetEquations=on  FunctionEvalNumThread=1  LocalSolverSampleTime=0.01  DoFixedCost=off  MaxNonlinIter=3  MaxModeIter=2  ComputeImpulses=off  ImpulseIterations=2  LinearAlgebra=auto  LinearAlgebraNumThread=0  EquationFormulation=NE_TIME_EF  DelaysMemoryBudget=1024  AutomaticFiltering=on  FilteringTimeConstant=0.001  PartitionStorageMethod=AS_NEEDED  PartitionMemoryBudget=1024  PartitionMethod=ROBUST  MultibodyUseLocalSolver=off  MultibodyLocalSolverChoice=ODE1  MultibodyLocalSolverSampleTime=0.001
  Speed Different : Sum  Inputs=+-
  Square1 : Math  Operator=square
  Stop Simulation1 : Stop
  Sum : Sum  Inputs=|+-
  Switch1 : Switch  Criteria=u2 ~= 0  SaturateOnIntegerOverflow=off  InputSameDT=off
  Terminator{,6..10} (6 alike) : Terminator
  Unit Conversion4 : UnitConversion
  V_pack1 : Gain  Gain=18
  Accel[ms2] : Outport
  Speed[ms] : Outport  Port=2
  Position[m] : Outport  Port=3
  SOC_SIM : Outport  Port=4
  wires:
  Discrete-Time Integrator1/1 -> Sum/1, Position[m]/1
  From Workspace9/1 -> Divide15/2
  Divide15/1 -> Discrete-Time Integrator/1, Accel[ms2]/1  "Veh_acceleartion"
  pos_follow/1 -> Sum/2
  Discrete-Time Integrator/1 -> Signal Specification4/1
  Signal Specification4/1 -> Discrete-Time Integrator1/1, Speed[ms]/1, [Speed_ms]
  PID Controller/1 -> Brake[%]1/1, Accel[%]1/1  "Acceleration"
  Speed Different/1 -> PID Controller/1  "Speed Different"
  Target speed/1 -> Speed Different/1
  vel_ego/1 -> Gain1/1
  Sum/1 -> [IVD]
  Divide28/1 -> Divide29/1
  From Workspace20/1 -> Divide34/2
  Add1/1 -> Divide33/1
  [T_motor] -> Divide38/1
  Divide29/1 -> [T_motor]
  Signal Specification9/1 -> [Motor_radpsec]
  [IVD] -> Saturation1/1
  Gain20/1 -> [Motor_RPM]
  Add13/1 -> Divide25/1
  Divide39/1 -> [Electric_Power]
  Add14/1 -> [F_accel]
  [Speed_ms] -> Divide22/2
  [F_resistance] -> Add11/2
  Divide1/1 -> Add1/2  "Motor_Torque[N.m]"
  From Workspace14/1 -> Divide29/2
  Divide23/1 -> Gain/1  "F_aero"
  Brake[%]1/1 -> Divide25/2, Divide2/1
  Unit Conversion4/1 -> Signal Specification9/1
  From Workspace21/1 -> Divide35/3
  Divide35/1 -> Divide36/2
  [Motor_RPM] -> 2-D Lookup Table1/1
  Gain23/1 -> Divide39/2
  Compare To Constant3/1 -> Switch1/2
  Divide37/1 -> Gain20/1
  Divide34/1 -> Add14/2
  BPP[%]*MAX_Brake_Force[N]1/1 -> Add14/1  "Brake_Force"
  From Workspace/1 -> Divide23/3
  From Workspace22/1 -> Divide37/2
  Constant9/1 -> Divide35/1
  [Motor_efficiency] -> Gain23/1
  Constant10/1 -> Divide35/2
  [Speed_ms] -> Square1/1
  Add11/1 -> Divide28/1
  Square1/1 -> Divide23/2
  2-D Lookup Table1/1 -> [Motor_efficiency]
  Gain14/1 -> BPP[%]*MAX_Brake_Force[N]1/1
  From Workspace19/1 -> Add13/2
  Add15/1 -> [F_resistance]
  Friction_Loss1/1 -> Divide22/1
  [Motor_RPM] -> Signal Specification8/1
  Drag coefficient1/1(C_drag) -> Divide23/1
  [Motor_radpsec] -> Divide38/2
  From Workspace1/1 -> Divide2/2
  Accel[%]1/1 -> Accel1/1
  Constant8/1 -> Add13/1
  Divide36/1 -> Divide37/1
  [Motor_Power] -> Divide39/1
  MAX Torque1/1 -> Divide27/2, Divide1/1
  Accel1/1 -> Divide1/2
  Divide33/1 -> Divide34/1
  [F_accel] -> Add11/1
  [T_motor] -> 2-D Lookup Table1/2
  Rolling_Loss1/1 -> Divide3/1
  Divide27/1 -> Add1/1  "Motor_Torque[N.m]"
  Saturation1/1 -> Drag coefficient1/1(IVD)
  Switch1/1 -> Add15/1  "F_rolling"
  From Workspace15/1 -> Divide28/2
  Gain13/1 -> Divide27/1
  Constant3/1 -> Switch1/3
  Divide25/1 -> Gain14/1
  Divide22/1 -> Add15/2  "F_friction"
  Divide2/1 -> Gain13/1
  Divide38/1 -> [Motor_Power]
  [Motor_RPM] -> MAX Torque1/1
  Signal Specification8/1 -> Unit Conversion4/1
  From Workspace18/1 -> Divide33/2
  [Speed_ms] -> Divide36/1
  [F_accel] -> Divide15/1
  [Speed_ms] -> Compare To Constant3/1
  Gain/1 -> Add15/3
  From Workspace2/1 -> Divide23/4
  From Workspace3/1 -> Divide3/2
  From Workspace4/1 -> Divide3/3
  Divide3/1 -> Switch1/1  "F_aero"
  Gain1/1 -> Speed Different/2
  pos_ego/1 -> Terminator/1
  NewPack1/5(vCell) -> Terminator8/1
  SOC2OCV Table/1 -> V_pack1/1  "Vsoc"
  SOC2R0 Table/1 -> MATLAB Function/3(R0)
  NewPack1/3(socCell) -> SOC_SIM/1, Gain3/1  "SOC_LV"
  Compare To Constant1/1 -> Stop Simulation1/1
  NewPack1/4(socParallelAssembly) -> Terminator10/1
  Gain3/1 -> Compare To Constant1/1
  MATLAB Function/1(I) -> Simulink-PS Converter1/1  "Current_pack"
  NewPack1/2(numCyclesCell) -> Terminator7/1
  V_pack1/1 -> MATLAB Function/2(OCV)
  soc_ego/1 -> SOC2R0 Table/1, SOC2OCV Table/1
  NewPack1/6(vParallelAssembly) -> Terminator9/1
  [Electric_Power] -> MATLAB Function/1(P)
  NewPack1/1(iCell) -> Terminator6/1
  connections:
  Solver Configuration1/RConn1 -- Controlled Current Source1/RConn2 -- Electrical Reference1/LConn1 -- NewPack1/LConn1
  Simulink-PS Converter1/RConn1 -- Controlled Current Source1/RConn1
  NewPack1/RConn1 -- Controlled Current Source1/LConn1
